simulink model "castor_extras"  (R2020b)
settings: Solver=VariableStepAuto  StartTime=0.0  StopTime=300  MaxStep=0.01  RelTol=1e-3
libraries: pid_lib x1, simulink x1
settings Model: Creator=Daniel  LastModifiedBy=Daniel
settings DebuggingCC: SFMachineParentedDataDiag=error

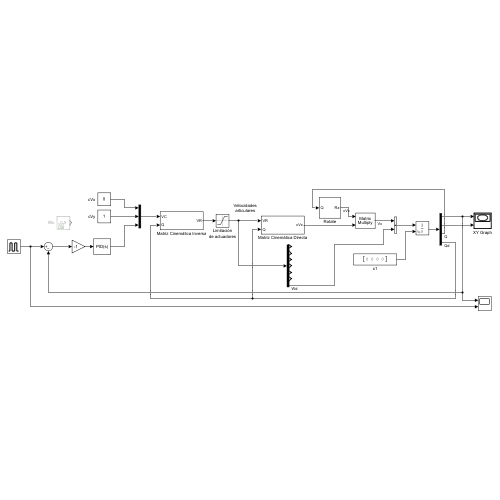
[thumbnail: Simulink's stored preview of the top-level diagram]
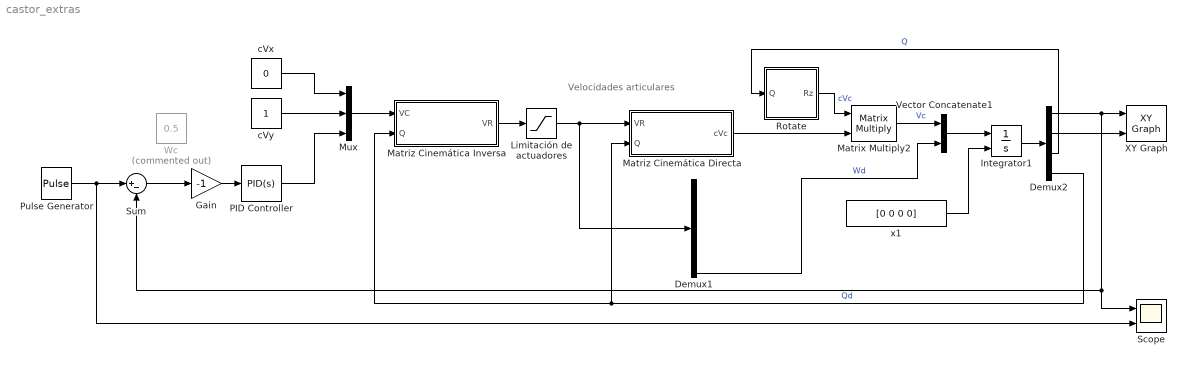
== system castor_extras ==
  note: Velocidades
      | articulares
  Demux1 : Demux  Outputs=7
  Demux2 : Demux
  Gain : Gain  Gain=-1
  Integrator1 : Integrator  InitialConditionSource=external
  Limitación de actuadores : Saturate  UpperLimit=1.5  LowerLimit=-1.5
  Matrix Multiply2 : Product  Multiplication=Matrix(*)
  Matriz Cinemática Directa : Subsystem  mask{d1=0.05, d2=0.05, d3=0.05, d4=0.05}
      mask prompts: d1 "Traction Wheel1 Offset"; d2 "Traction Wheel2 Offset"; d3 "Steering Offset"; d4 "Steering Length"
  Matriz Cinemática Inversa : Subsystem  mask{d1=0.05, d2=0.05, d3=0.05, d4=0.05}
      mask prompts: d1 "Traction Wheel1 Offset"; d2 "Traction Wheel2 Offset"; d3 "Steering Offset"; d4 "Steering Length"
  Mux : Mux  Inputs=3
  PID Controller : pid_lib/PID Controller  Controller=PID  Form=Parallel  TimeDomain=Continuous-time  UseExternalTs=off  SampleTime=-1  IntegratorMethod=Forward Euler  FilterMethod=Forward Euler  ControllerParametersSource=internal  P=0.1  I=0.01  D=1  UseFilter=on  N=100  TunerSelectOption=Transfer Function Based (PID Tuner App)  InitialConditionSource=internal  InitialConditionForIntegrator=0  InitialConditionForFilter=0  DifferentiatorICPrevScaledInput=0  ExternalReset=none  TrackingMode=off  Kt=1  LimitOutput=off  SatLimitsSource=internal  UpperSaturationLimit=inf  LowerSaturationLimit=-inf  LinearizeAsGain=on  AntiWindupMode=none  Kb=1  POutMin=[]  POutMax=[]  IOutMin=[]  IOutMax=[]  DOutMin=[]  DOutMax=[]  NOutMin=[]  NOutMax=[]  SumOutMin=[]  SumOutMax=[]  SaturationOutMin=[]  SaturationOutMax=[]  PParamMin=[]  PParamMax=[]  IParamMin=[]  IParamMax=[]  DParamMin=[]  DParamMax=[]  NParamMin=[]  NParamMax=[]  KbParamMin=[]  KbParamMax=[]  KtParamMin=[]  KtParamMax=[]  KbOutMin=[]  KbOutMax=[]  KtOutMin=[]  KtOutMax=[]  IntegratorOutMin=[]  IntegratorOutMax=[]  FilterOutMin=[]  FilterOutMax=[]  SumI1OutMin=[]  SumI1OutMax=[]  SumI2OutMin=[]  SumI2OutMax=[]  SumI3OutMin=[]  SumI3OutMax=[]  SumI4OutMin=[]  SumI4OutMax=[]  SumDOutMin=[]  SumDOutMax=[]  DifferentiatorOutMin=[]  DifferentiatorOutMax=[]  FilterDiffOutCoefMin=[]  FilterDiffOutCoefMax=[]  ReciprocalOutMin=[]  ReciprocalOutMax=[]  SumDenOutMin=[]  SumDenOutMax=[]  SumNumOutMin=[]  SumNumOutMax=[]  DivideOutMin=[]  DivideOutMax=[]  UdiffTsProdOutMin=[]  UdiffTsProdOutMax=[]  NTsProdOutMin=[]  NTsProdOutMax=[]  UintegralTsProdOutMin=[]  UintegralTsProdOutMax=[]  UngainTsProdOutMin=[]  UngainTsProdOutMax=[]  IntegratorContinuousStateAttributes=''  IntegratorStateMustResolveToSignalObject=off  IntegratorRTWStateStorageClass=Auto  FilterContinuousStateAttributes=''  FilterStateMustResolveToSignalObject=off  FilterRTWStateStorageClass=Auto  ParallelPVariant=InternalParameters  IdealPVariant=Disabled  IVariant=InternalParameters  DVariant=InternalParameters  IntegratorVariant=Continuous  SatVariant=Disabled  AWVariant=Passthrough  PCopyVariant=Disabled  TRVariant=Disabled  FdbkBlocksVariant=Forward  IdealPFdbkVariant=Disabled  SatFdbkVariant=Disabled  DerivativeFilterVariant=ContFilter  NVariant=InternalParameters  NCopyVariant=Disabled  FilterICVariant=InternalICsFilter  IntegratorICVariant=InternalICs  ExternalResetVariant=Disabled  TRSumVariant=Passthrough  SumFdbkVariant=Disabled  SumVariant=Sum_PID  TsampFilterVariant=InternalTs  TsampNgainVariant=Passthrough  TsampIntegralVariant=Passthrough  ExternalSaturationOutDataTypeStr=Inherit: Same as second input
  Pulse Generator : DiscretePulseGenerator  PulseType=Time based  Period=50  PulseWidth=50
  Rotate : Subsystem
  Scope : Scope  NumInputPorts=2
  Sum : Sum  Inputs=|+-
  Vector Concatenate1 : Concatenate
  Wc : Constant  Commented=on  Value=0.5
  XY Graph : simulink/Sinks/XY Graph  xmin=-1  xmax=1  ymin=-1  ymax=1  st=-1
  cVx : Constant  Value=0
  cVy : Constant
  x1 : Constant  Value=[0 0 0 0]  SampleTime=-1
  wires:
  cVy/1 -> Mux/2
  cVx/1 -> Mux/1
  Demux1/7 -> Vector Concatenate1/2  "Wd"
  Matriz Cinemática Directa/1(cVc) -> Matrix Multiply2/2
  Rotate/1(Rz) -> Matrix Multiply2/1  "cVc"
  Matrix Multiply2/1 -> Vector Concatenate1/1  "Vc"
  Vector Concatenate1/1 -> Integrator1/1
  x1/1 -> Integrator1/2
  Integrator1/1 -> Demux2/1
  Demux2/1 -> Sum/2, Scope/1, XY Graph/1
  Demux2/2 -> XY Graph/2
  Mux/1 -> Matriz Cinemática Inversa/1(VC)
  Demux2/3 -> Rotate/1(Q)  "Q"
  Limitación de actuadores/1 -> Demux1/1, Matriz Cinemática Directa/1(VR)
  Demux2/4 -> Matriz Cinemática Directa/2(Q), Matriz Cinemática Inversa/2(Q)  "Qd"
  PID Controller/1 -> Mux/3
  Gain/1 -> PID Controller/1
  Sum/1 -> Gain/1
  Pulse Generator/1 -> Scope/2, Sum/1
  Matriz Cinemática Inversa/1(VR) -> Limitación de actuadores/1

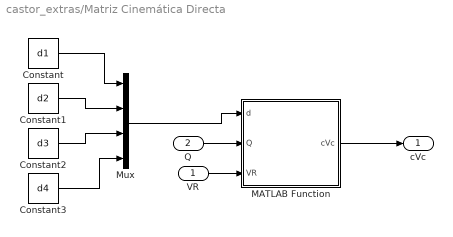
== system castor_extras/Matriz Cinemática Directa ==
  VR : Inport
  Q : Inport  Port=2
  Constant : Constant  Value=d1
  Constant1 : Constant  Value=d2
  Constant2 : Constant  Value=d3
  Constant3 : Constant  Value=d4
  MATLAB Function : MATLAB Function  TreatAsAtomicUnit=on
  Mux : Mux
  cVc : Outport
  wires:
  VR/1 -> MATLAB Function/3(VR)
  MATLAB Function/1(cVc) -> cVc/1
  Constant1/1 -> Mux/2
  Constant2/1 -> Mux/3
  Constant/1 -> Mux/1
  Constant3/1 -> Mux/4
  Mux/1 -> MATLAB Function/1(d)
  Q/1 -> MATLAB Function/2(Q)

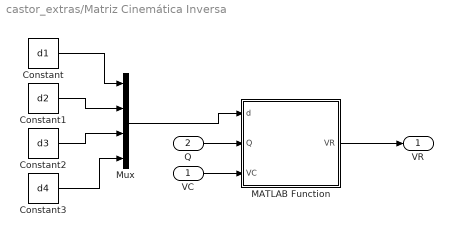
== system castor_extras/Matriz Cinemática Inversa ==
  VC : Inport
  Q : Inport  Port=2
  Constant : Constant  Value=d1
  Constant1 : Constant  Value=d2
  Constant2 : Constant  Value=d3
  Constant3 : Constant  Value=d4
  MATLAB Function : MATLAB Function  TreatAsAtomicUnit=on
  Mux : Mux
  VR : Outport
  wires:
  Q/1 -> MATLAB Function/2(Q)
  MATLAB Function/1(VR) -> VR/1
  Constant1/1 -> Mux/2
  Constant2/1 -> Mux/3
  Constant/1 -> Mux/1
  Constant3/1 -> Mux/4
  Mux/1 -> MATLAB Function/1(d)
  VC/1 -> MATLAB Function/3(VC)

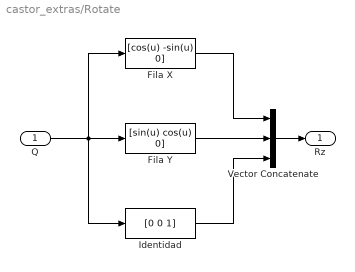
== system castor_extras/Rotate ==
  Q : Inport
  Fila X : MATLABFcn  MATLABFcn=[cos(u) -sin(u) 0]  OutputDimensions=[1 3]  Output1D=off
  Fila Y : MATLABFcn  MATLABFcn=[sin(u) cos(u) 0]  OutputDimensions=[1 3]  Output1D=off
  Identidad : MATLABFcn  MATLABFcn=[0 0 1]  OutputDimensions=[1 3]  Output1D=off
  Vector Concatenate : Concatenate  NumInputs=3  Mode=Multidimensional array
  Rz : Outport
  wires:
  Q/1 -> Identidad/1, Fila Y/1, Fila X/1
  Vector Concatenate/1 -> Rz/1
  Fila Y/1 -> Vector Concatenate/2
  Fila X/1 -> Vector Concatenate/1
  Identidad/1 -> Vector Concatenate/3

== matlab function castor_extras/Matriz Cinemática Directa/MATLAB Function ==
  data: d input; Q input; cVc output; VR input
function cVc = fcn(d,Q,VR)

    J1 = [0 0; 1 d(1); 0 1];
    J2 = [0 0; 1 -d(2); 0 1];
    J3 = [-sin(Q) -d(4)*cos(Q)-d(3) d(3); cos(Q) -d(4)*sin(Q) 0; 0 1 -1];
    
    A=[eye(3); eye(3); eye(3)];
    B=[J1 zeros(3,2) zeros(3,3); zeros(3,2) J2 zeros(3,3); zeros(3,2) zeros(3,2) J3];

    cVc = inv(A'*A)*A'*B*VR;

end

== matlab function castor_extras/Matriz Cinemática Inversa/MATLAB Function ==
  data: d input; VR output; Q input; VC input
function VR = fcn(d,Q,VC)

    J1 = [0 0; 1 d(1); 0 1];
    J2 = [0 0; 1 -d(2); 0 1];
    J3 = [-sin(Q) -d(4)*cos(Q)-d(3) d(3); cos(Q) -d(4)*sin(Q) 0; 0 1 -1];
    
    % Creación de las matrices A y Jacobiana
    A=[eye(3); eye(3); eye(3)];
    B=[J1 zeros(3,2) zeros(3,3); zeros(3,2) J2 zeros(3,3); zeros(3,2) zeros(3,2) J3];

    VR = inv(B'*B)*B'*A*VC;

end
